simulink model "DegradationParameterVResistor"  (R2021a)
settings: Solver=VariableStepAuto  StartTime=0.0  StopTime=10.0  RelTol=1e-3
undefined symbols (not defined in the file or in its folder): Vres_resistance_adjustment
libraries: PB_Library_Master_Working x2
settings Model: Creator=sfaulk  LastModifiedBy=sfaulk

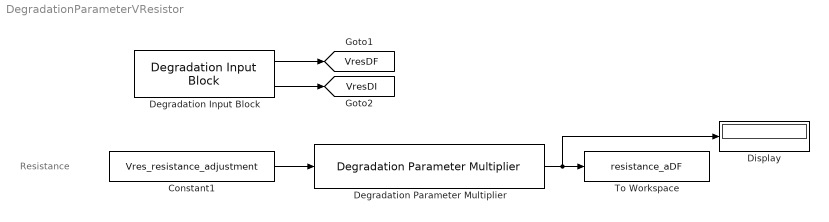
== system DegradationParameterVResistor ==
  note: Resistance
  Constant1 : Constant  Value=Vres_resistance_adjustment
  Degradation Input Block : PB_Library_Master_Working/Degradation Input Block  SystemSampleTime=-1  VariantActivationTime=update diagram  Latency=0  AutoFrameSizeCalculation=off
      link override Degradation Input Value: Value=Vres_degradation_input
  Degradation Parameter Multiplier : PB_Library_Master_Working/Degradation Parameter Multiplier  SystemSampleTime=-1  VariantActivationTime=update diagram  Latency=0  AutoFrameSizeCalculation=off
      link override From14: GotoTag=VresDF
      link override From15: GotoTag=VresDI
  Display : Display
  To Workspace : ToWorkspace  VariableName=resistance_aDF  SaveFormat=Timeseries  SampleTime=-1
      settings: Save2DSignal=2-D array (concatenate along first dimension)
  tag scope: VresDF=global, VresDI=global
  wires:
  Constant1/1 -> Degradation Parameter Multiplier/1
  Degradation Parameter Multiplier/1 -> Display/1, To Workspace/1
  Degradation Input Block/2 -> [VresDI]
  Degradation Input Block/1 -> [VresDF]
